simulink model "HeadwayControlR2017a"  (R2017a)
settings: Solver=ode45  StartTime=0.0  StopTime=tsim  MaxStep=.1  RelTol=1e-3
values from neighbouring files (symbols this model uses):
  EndVel = (Time2-Time1)*Slope+StartVel    (= 31.525)    [HeadwayControlSimScript.m]    (also in HeadwayControlSimScriptExperiment.m; HeadwayControlSimScriptSimplified.m)
  h = 2    [HeadwayControlSimScript.m]    (also in HeadwayControlSimScriptExperiment.m; HeadwayControlSimScriptSimplified.m)
  InputNum = 3    [HeadwayControlSimScript.m]    (also in HeadwayControlSimScriptExperiment.m; HeadwayControlSimScriptSimplified.m)
  InputTime = 1    [HeadwayControlSimScript.m]    (also in HeadwayControlSimScriptExperiment.m; HeadwayControlSimScriptSimplified.m)
  lambda = 0.001    [HeadwayControlSimScript.m]    (also in HeadwayControlSimScriptExperiment.m = 0.135; HeadwayControlSimScriptSimplified.m)
  Slope = 0.5*g    (= 4.905)    [HeadwayControlSimScript.m]    (also in HeadwayControlSimScriptExperiment.m; HeadwayControlSimScriptSimplified.m)
  StartVel = 7    [HeadwayControlSimScript.m]    (also in HeadwayControlSimScriptExperiment.m; HeadwayControlSimScriptSimplified.m)
  tau = .5    (= 0.5)    [HeadwayControlSimScript.m]    (also in HeadwayControlSimScriptExperiment.m; HeadwayControlSimScriptSimplified.m)
  Time1 = 2    [HeadwayControlSimScript.m]    (also in HeadwayControlSimScriptExperiment.m = 35; HeadwayControlSimScriptSimplified.m)
  Time2 = Time1 + DTime    (= 7)    [HeadwayControlSimScript.m]    (also in HeadwayControlSimScriptExperiment.m = 40; HeadwayControlSimScriptSimplified.m)
undefined symbols (not defined in the file or in its folder): heaviside
libraries: simulink x2
settings Model: Creator=domin  LastModifiedBy=domin

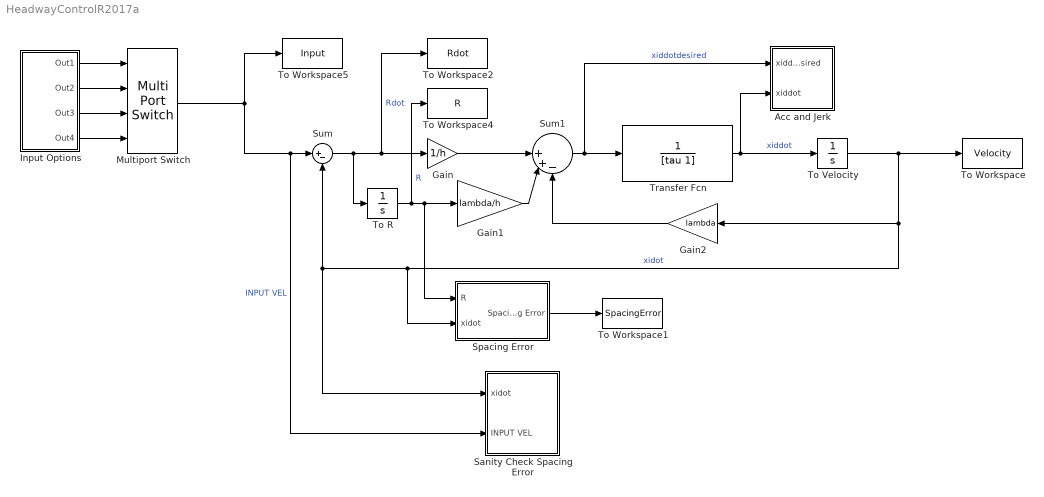
== system HeadwayControlR2017a ==
  Acc and Jerk : Subsystem
  Gain : Gain  Gain=1/h
  Gain1 : Gain  Gain=lambda/h
  Gain2 : Gain  Gain=lambda
  Input Options : Subsystem
  Multiport Switch : MultiPortSwitch
  Sanity Check Spacing Error : Subsystem
  Spacing Error : Subsystem
  Sum : Sum  Inputs=|+-
  Sum1 : Sum  Inputs=||++-
  To R : Integrator  InitialCondition=h*StartVel
  To Velocity : Integrator  InitialCondition=StartVel
  To Workspace : ToWorkspace  VariableName=Velocity  SampleTime=-1
  To Workspace1 : ToWorkspace  VariableName=SpacingError  SampleTime=-1
  To Workspace2 : ToWorkspace  VariableName=Rdot  SampleTime=-1
  To Workspace4 : ToWorkspace  VariableName=R  SampleTime=-1
  To Workspace5 : ToWorkspace  VariableName=Input  SampleTime=-1
  Transfer Fcn : TransferFcn  Denominator=[tau 1]
  wires:
  Sum/1 -> To R/1, To Workspace2/1, Gain/1  "Rdot"
  To R/1 -> To Workspace4/1, Spacing Error/1(R), Gain1/1  "R"
  Gain/1 -> Sum1/1
  Gain1/1 -> Sum1/2
  Sum1/1 -> Acc and Jerk/1(xiddotdesired), Transfer Fcn/1  "xiddotdesired"
  Transfer Fcn/1 -> Acc and Jerk/2(xiddot), To Velocity/1  "xiddot"
  To Velocity/1 -> Spacing Error/2(xidot), Sum/2, Sanity Check Spacing Error/1(xidot), Gain2/1, To Workspace/1  "xidot"
  Gain2/1 -> Sum1/3
  Multiport Switch/1 -> To Workspace5/1, Sum/1, Sanity Check Spacing Error/2(INPUT VEL)  "INPUT VEL"
  Input Options/1(Out1) -> Multiport Switch/1
  Input Options/2(Out2) -> Multiport Switch/2
  Input Options/3(Out3) -> Multiport Switch/3
  Input Options/4(Out4) -> Multiport Switch/4
  Spacing Error/1(Spacing Error) -> To Workspace1/1

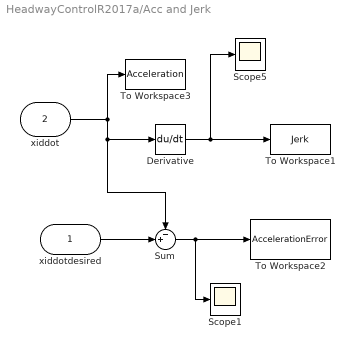
== system HeadwayControlR2017a/Acc and Jerk ==
  xiddotdesired : Inport
  xiddot : Inport  Port=2
  Derivative : Derivative
  Scope1 : Scope
  Scope5 : Scope
  Sum : Sum  Inputs=-+|
  To Workspace1 : ToWorkspace  VariableName=Jerk  SampleTime=-1
  To Workspace2 : ToWorkspace  VariableName=AccelerationError  SampleTime=-1
  To Workspace3 : ToWorkspace  VariableName=Acceleration  SampleTime=-1
  wires:
  xiddot/1 -> To Workspace3/1, Derivative/1, Sum/1
  Derivative/1 -> To Workspace1/1, Scope5/1
  xiddotdesired/1 -> Sum/2
  Sum/1 -> Scope1/1, To Workspace2/1

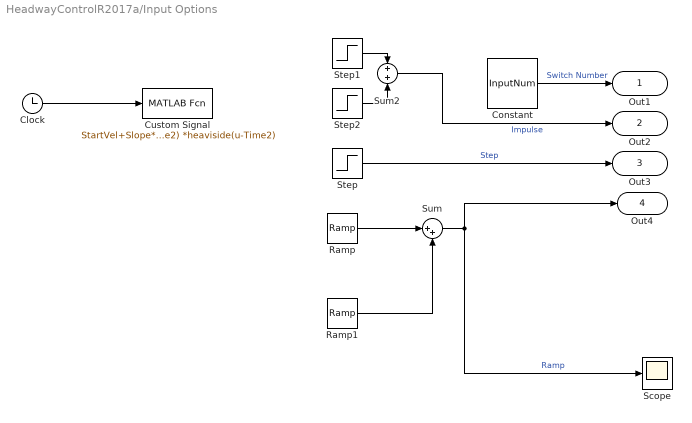
== system HeadwayControlR2017a/Input Options ==
  Clock : Clock
  Constant : Constant  Value=InputNum
  Custom Signal : MATLABFcn  MATLABFcn=StartVel+Slope*(u-Time1) *heaviside(u-Time1)-Slope*(u-Time2) *heaviside(u-Time2)  OutputDimensions=1
  Ramp : simulink/Sources/Ramp  slope=Slope  start=Time1  X0=StartVel
  Ramp1 : simulink/Sources/Ramp  slope=-Slope  start=Time2  X0=0
  Scope : Scope
  Step : Step  Time=InputTime  Before=StartVel  After=EndVel  SampleTime=0
  Step1 : Step  Time=InputTime  Before=StartVel  After=StartVel+(1*10^10)  SampleTime=0
  Step2 : Step  Time=InputTime + (1*10^-10)  After=-(1*10^10)  SampleTime=0
  Sum : Sum  Inputs=|++
  Sum2 : Sum
  Out1 : Outport
  Out2 : Outport  Port=2
  Out3 : Outport  Port=3
  Out4 : Outport  Port=4
  wires:
  Clock/1 -> Custom Signal/1
  Sum2/1 -> Out2/1  "Impulse"
  Constant/1 -> Out1/1  "Switch Number"
  Step2/1 -> Sum2/2
  Step1/1 -> Sum2/1
  Step/1 -> Out3/1  "Step"
  Ramp/1 -> Sum/1
  Ramp1/1 -> Sum/2
  Sum/1 -> Out4/1, Scope/1  "Ramp"

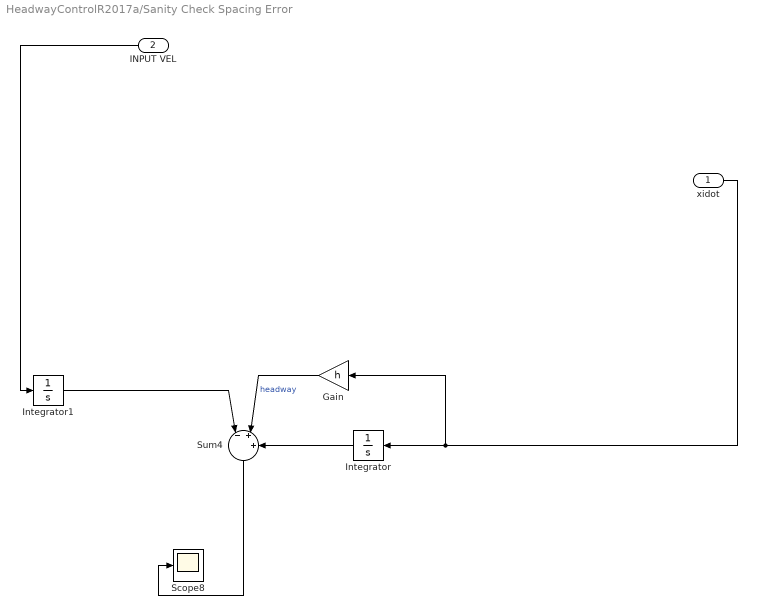
== system HeadwayControlR2017a/Sanity Check Spacing Error ==
  xidot : Inport
  INPUT VEL : Inport  Port=2
  Gain : Gain  Gain=h
  Integrator : Integrator
  Integrator1 : Integrator  InitialCondition=h*StartVel
  Scope8 : Scope
  Sum4 : Sum  Inputs=|-++
  wires:
  Integrator/1 -> Sum4/3
  Integrator1/1 -> Sum4/1
  xidot/1 -> Gain/1, Integrator/1
  INPUT VEL/1 -> Integrator1/1
  Sum4/1 -> Scope8/1
  Gain/1 -> Sum4/2  "headway"

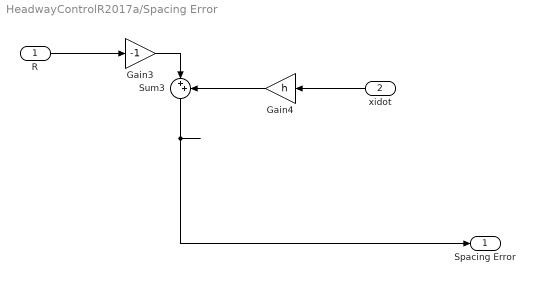
== system HeadwayControlR2017a/Spacing Error ==
  R : Inport
  xidot : Inport  Port=2
  Gain3 : Gain  Gain=-1
  Gain4 : Gain  Gain=h
  Sum3 : Sum  Inputs=|++
  Spacing Error : Outport
  wires:
  Sum3/1 -> Spacing Error/1
  R/1 -> Gain3/1
  xidot/1 -> Gain4/1
  Gain3/1 -> Sum3/1
  Gain4/1 -> Sum3/2
